simulink model "tetherNnode_th"  (R2018b)
settings: Solver=VariableStepAuto  StartTime=0.0  StopTime=sim_time  MaxStep=dt  RelTol=1e-3
values from neighbouring files (symbols this model uses):
  flow = [0;0;0]    [tetherNnode_ts.m]
  numTethers = 3    [tetherNnode_ts.m]
libraries: tetherNnode_ul x1
settings Model: Creator=asiddiq2  LastModifiedBy=asiddiq2

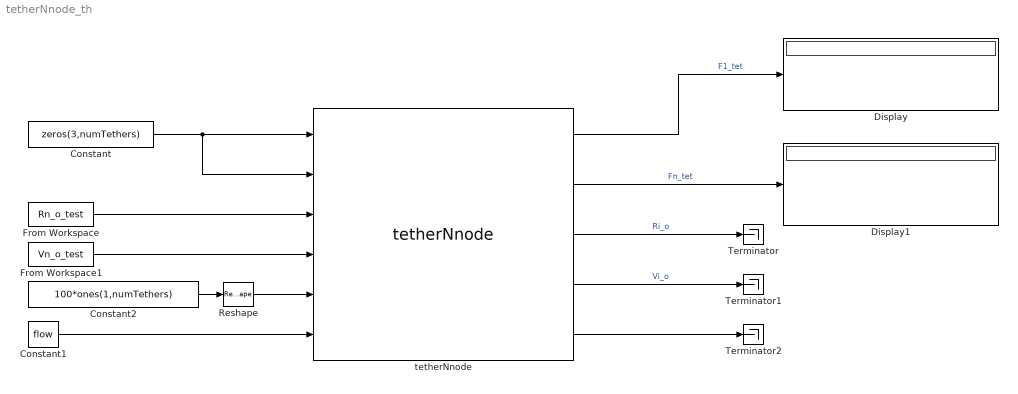
== system tetherNnode_th ==
  Constant : Constant  Value=zeros(3,numTethers)  VectorParams1D=off
  Constant1 : Constant  Value=flow  VectorParams1D=off
  Constant2 : Constant  Value=100*ones(1,numTethers)  VectorParams1D=off
  Display : Display
  Display1 : Display
  From Workspace : FromWorkspace  VariableName=Rn_o_test  SampleTime=0
  From Workspace1 : FromWorkspace  VariableName=Vn_o_test  SampleTime=0
  Reshape : Reshape  OutputDimensionality=Row vector (2-D)
  Terminator : Terminator
  Terminator1 : Terminator
  Terminator2 : Terminator
  tetherNnode : tetherNnode_ul/tetherNnode  gravAccl=grav  rhoFluid=rho_fluid  massBdy=mass  numNode=thr.numNodes.Value  thrDia=thr.thrDiameter.Value  thrRho=thr.thrDensity.Value  thrYoungs=thr.thrYoungs.Value  thrZeta=thr.thrDampingRatio.Value  thrCd=thr.thrDragCoeff.Value
  wires:
  tetherNnode/1 -> Display/1  "F1_tet"
  tetherNnode/4 -> Terminator1/1  "Vi_o"
  tetherNnode/3 -> Terminator/1  "Ri_o"
  tetherNnode/2 -> Display1/1  "Fn_tet"
  tetherNnode/5 -> Terminator2/1
  From Workspace1/1 -> tetherNnode/4
  Constant1/1 -> tetherNnode/6
  Constant2/1 -> Reshape/1
  From Workspace/1 -> tetherNnode/3
  Constant/1 -> tetherNnode/2, tetherNnode/1
  Reshape/1 -> tetherNnode/5
